simulink subsystem "phi_r_observer_voltage"  (R2022b)
settings: Solver=VariableStepAuto  StartTime=0.0  StopTime=10.0  RelTol=1e-3
undefined symbols (not defined in the file or in its folder): K7, K8, K9
settings Model: Creator=jack  LastModifiedBy=jack

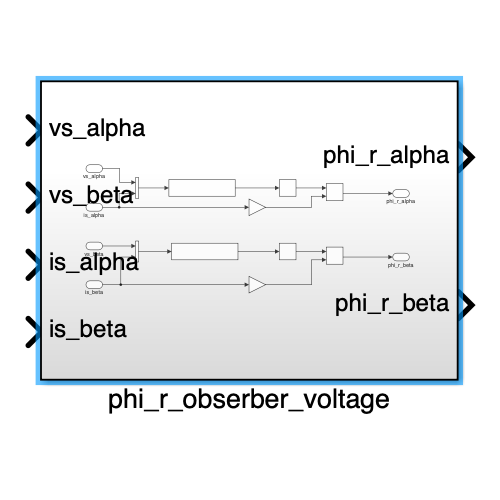
[thumbnail: Simulink's stored preview of the top-level diagram]
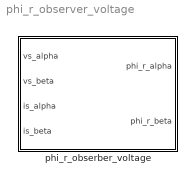
== system phi_r_observer_voltage ==
  phi_r_obserber_voltage : Subsystem

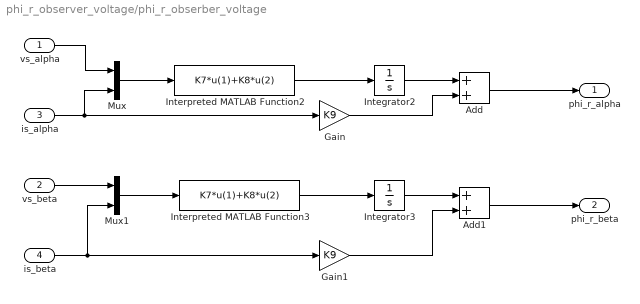
== system phi_r_observer_voltage/phi_r_obserber_voltage ==
  vs_alpha : Inport
  vs_beta : Inport  Port=2
  is_alpha : Inport  Port=3
  is_beta : Inport  Port=4
  Add : Sum
  Add1 : Sum
  Gain : Gain  Gain=K9
  Gain1 : Gain  Gain=K9
  Integrator2 : Integrator
  Integrator3 : Integrator
  Interpreted MATLAB Function2 : MATLABFcn  MATLABFcn=K7*u(1)+K8*u(2)
  Interpreted MATLAB Function3 : MATLABFcn  MATLABFcn=K7*u(1)+K8*u(2)
  Mux : Mux  Inputs=2
  Mux1 : Mux  Inputs=2
  phi_r_alpha : Outport
  phi_r_beta : Outport  Port=2
  wires:
  Interpreted MATLAB Function2/1 -> Integrator2/1
  Interpreted MATLAB Function3/1 -> Integrator3/1
  vs_alpha/1 -> Mux/1
  is_alpha/1 -> Gain/1, Mux/2
  Mux/1 -> Interpreted MATLAB Function2/1
  Integrator2/1 -> Add/1
  Add/1 -> phi_r_alpha/1
  Gain/1 -> Add/2
  Integrator3/1 -> Add1/1
  Add1/1 -> phi_r_beta/1
  is_beta/1 -> Mux1/2, Gain1/1
  vs_beta/1 -> Mux1/1
  Mux1/1 -> Interpreted MATLAB Function3/1
  Gain1/1 -> Add1/2
